simulink model "main"  (R2025a)
settings: Solver=VariableStepAuto  StartTime=0.0  StopTime=20  RelTol=1e-3
model workspace (MAT data in the model file):
  AccelNoise = [6.4e-07 6.4e-07 6.4e-07]
  AccelSampleTime = 0.001
  BaroSampleTime = 0.02
  BurnTime = 3.5
  GPSSampleTime = 0.06
  GimbalDelay = 0.02
  GimbalMaxRate = 5
  GimbalMaxSkew = 0.0872665
  Gravity = 9.81
  GyroNoise = [1.1e-08 1.1e-08 1.1e-08]
  GyroSampleTime = 0.001
  IMULocation = [0 0 0]
  InitialCG = [0 0 0]
  Mass = 1
  MaxAttitudeSetpoint = 0.15
  MaxThrust = 25
  MinThrust = 12
  MomentArm = 0.28
  RocketImpulse = 49.6
  RotationMatrix = [1  0  0; 0  1  0; 0  0  1]
  ServoSampleTime = 0.02
  Sig = Simulink.Signal
  Sig.Dimensions = -1
  Sig.DimensionsMode = 'auto'
  Sig.Complexity = 'auto'
  Sig.SampleTime = -1
  Sig.SamplingMode = 'auto'
  Sig.DataType = 'auto'
  Sig1 = Simulink.Signal
  Sig1.Dimensions = -1
  Sig1.DimensionsMode = 'auto'
  Sig1.Complexity = 'auto'
  Sig1.SampleTime = -1
  Sig1.SamplingMode = 'auto'
  Sig1.DataType = 'auto'
  VehicleMOI = [0.02  0  0; 0  0.1  0; 0  0  0.1]
  WheelDelay = 0.02
  WheelMOI = 0.0045
  WheelMaxAcceleration = 120
  WheelMaxRate = 500
  WheelSampleTime = 0.05
undefined symbols (not defined in the file): DiscIntNeverNeededParam
libraries: slpidlib x5, aerolibutil x4, aerolibnav x2, aerolibsim3d x2, sensorgpslib x1, sim3dlib x1, matrix_library x1
(part 1 of 2)
settings Model: Creator=jebid  LastModifiedBy=jebid

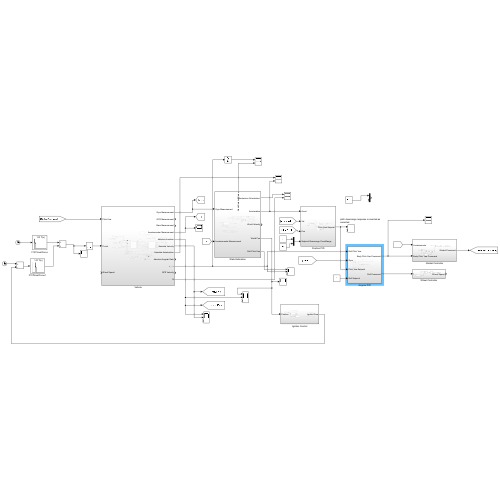
[thumbnail: Simulink's stored preview of the top-level diagram]
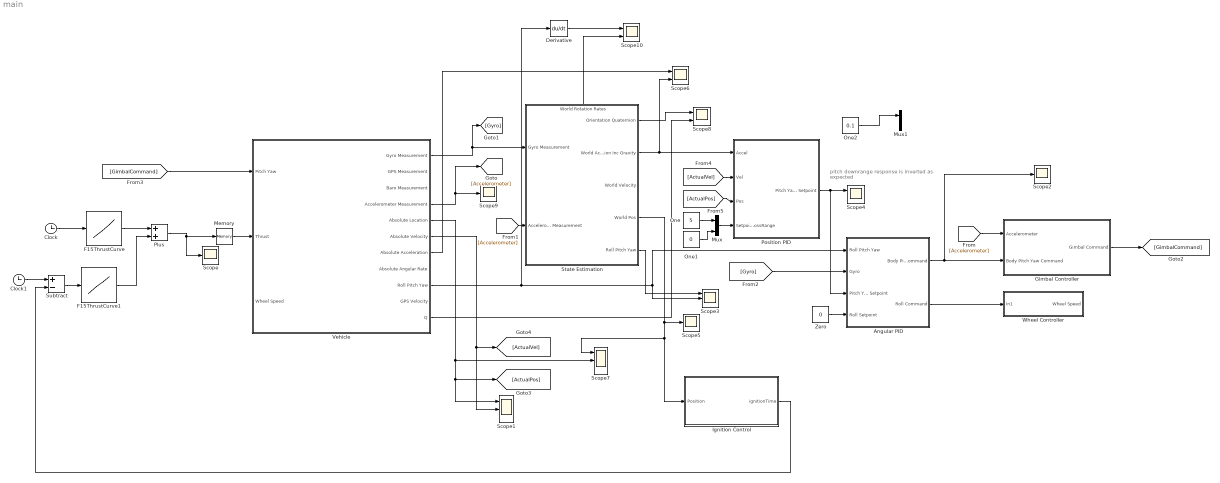
== system main ==
  note: pitch downrange response is inverted as expected
  Angular PID : Subsystem
  Clock : Clock
  Clock1 : Clock
  Derivative : Derivative
  F15ThrustCurve : Lookup_n-D  NumberOfTableDimensions=1  BreakpointsForDimension1=[0;0.14799999999999999;0.22800000000000001;0.29399999999999998;0.35299999999999998;0.38200000000000001;0.41899999999999998;0.47699999999999998;0.52000000000000002;0.59299999999999997;0.68799999999999994;0.85499999999999998;1.0369999999999999;1.2050000000000001;1.423;1.452;1.5029999999999999;1.736;1.9550000000000001;2.21;2.4940000000000002;2.7629999999999999;3.1200000000000001;3.3820000000000001;3.4039999999999999;3.4180000000000001;3.4500000000000002;30]  Table=[0;7.6379999999999999;12.253;16.390999999999998;20.210000000000001;22.756;25.260000000000002;23.074000000000002;20.844999999999999;19.093;17.5;16.225000000000001;15.427;14.948;14.627000000000001;15.741;14.785;14.622999999999999;14.303000000000001;14.141;13.819000000000001;13.337999999999999;13.334;13.013;9.3520000000000003;4.8949999999999996;0;0]  InternalRulePriority=Speed  RndMeth=Simplest
  F15ThrustCurve1 : Lookup_n-D  NumberOfTableDimensions=1  BreakpointsForDimension1=[-10;0;0.14799999999999999;0.22800000000000001;0.29399999999999998;0.35299999999999998;0.38200000000000001;0.41899999999999998;0.47699999999999998;0.52000000000000002;0.59299999999999997;0.68799999999999994;0.85499999999999998;1.0369999999999999;1.2050000000000001;1.423;1.452;1.5029999999999999;1.736;1.9550000000000001;2.21;2.4940000000000002;2.7629999999999999;3.1200000000000001;3.3820000000000001;3.4039999999999999;3.4180000000000001;3.4500000000000002;30]  Table=[0;0;7.6379999999999999;12.253;16.390999999999998;20.210000000000001;22.756;25.260000000000002;23.074000000000002;20.844999999999999;19.093;17.5;16.225000000000001;15.427;14.948;14.627000000000001;15.741;14.785;14.622999999999999;14.303000000000001;14.141;13.819000000000001;13.337999999999999;13.334;13.013;9.3520000000000003;4.8949999999999996;0;0]  InternalRulePriority=Speed  RndMeth=Simplest
  Gimbal Controller : Subsystem
  Ignition Control : Subsystem
  Memory : Memory
  Mux : Mux  Inputs=2
  Mux1 : Mux  Inputs=2
  One : Constant  Value=5  OutDataTypeStr=Inherit: Inherit via back propagation
  One1 : Constant  Value=0  OutDataTypeStr=Inherit: Inherit via back propagation
  One2 : Constant  Value=0.1  OutDataTypeStr=Inherit: Inherit via back propagation
  Plus : Sum
  Position PID : Subsystem
  Scope{,2,5,9} (4 alike) : Scope
      Scope settings: ActiveDisplayYMinimum=-50.736387173772314  ActiveDisplayYMaximum=31.586324733859495  DataLoggingVariableName=ScopeData4
      Scope2 settings: ActiveDisplayYMinimum=-0.14523916731500583  ActiveDisplayYMaximum=0.12648126595285003  DataLoggingVariableName=ScopeData6
      Scope5 settings: ActiveDisplayYMinimum=-31.391925729370655  ActiveDisplayYMaximum=52.800871093838978  DataLoggingVariableName=ScopeData8
      Scope9 settings: ActiveDisplayYMinimum=-1  ActiveDisplayYMaximum=1  DataLoggingVariableName=ScopeData27
  Scope1 : Scope  NumInputPorts=3
      settings: ActiveDisplayYMinimum=-22.683231133577891  ActiveDisplayYMaximum=11.292289740871924  DataLoggingVariableName=ScopeData5
  Scope{4,6,8,10} (4 alike) : Scope  NumInputPorts=2
      Scope10 settings: ActiveDisplayYMinimum=0.0077606363117146  ActiveDisplayYMaximum=0.18302244133274109  DataLoggingVariableName=ScopeData29
      Scope4 settings: ActiveDisplayYMinimum=-0.36702058756794975  ActiveDisplayYMaximum=0.56051213237813946  DataLoggingVariableName=ScopeData14
      Scope6 settings: ActiveDisplayYMinimum=-12.621728801475598  ActiveDisplayYMaximum=24.903102267700667  DataLoggingVariableName=ScopeData15
      Scope8 settings: ActiveDisplayYMinimum=0.705787790554492  ActiveDisplayYMaximum=0.96095471743838046  DataLoggingVariableName=ScopeData17
  Scope3 : Scope  NumInputPorts=3
      settings: ActiveDisplayYMinimum=-0.2363689882566378  ActiveDisplayYMaximum=0.3544136524668004  DataLoggingVariableName=ScopeData7
  Scope7 : Scope  NumInputPorts=3
      settings: ActiveDisplayYMinimum=-22.879561375629812  ActiveDisplayYMaximum=31.102735527921809  DataLoggingVariableName=ScopeData16
  State Estimation : Subsystem
      settings: PortSchema="{\"entries\":[{\"content\":{\"sides\":[{\"content\":{\"connectorIds\":[\"In1\",\"In2\"]},\"type\":\"ConnectorPlacement.EquallySpacedRectSide\",\"uuid\":\"2c2c3dca-e4ed-4564-ae6f-11a940ebc0d2\"},{\"content\":{\"connectorIds\":[\"Out1\",\"Out2\",\"Out3\",\"Out4\",\"Out5\"],\"side\":\"RIGHT\"},\"type\":\"ConnectorPlacement.EquallySpacedRectSide\",\"uuid\":\"8d125d98-ae45-4016-ae84-ebbc5244d165\"},{\"content\":{\"connectorIds\":[\"Out6\"],\"side\":\"TOP\"},\"type\":\"ConnectorPlacement.EquallySpacedRectSide\",\"uuid\":\"d438488b-91d6-49f1-8b44-fd6b40ea1e09\"}]},\"type\":\"ConnectorPlacement.EquallySpacedConnector\",\"uuid\":\"85e5d060-1813-434d-86b8-3131fa751346\"}],\"packageUris\":[\"http://schema.mathworks.com/mf0/Connector/R2020b\"],\"version\":\"1.0\"}"
  Subtract : Sum  Inputs=+-
  Vehicle : Subsystem
  Wheel Controller : Subsystem
  Zero : Constant  Value=0  OutDataTypeStr=Inherit: Inherit via back propagation
  wires:
  Clock/1 -> F15ThrustCurve/1
  Vehicle/1(Gyro Measurement) -> [Gyro], State Estimation/1(Gyro Measurement)
  State Estimation/4(World Pos) -> Scope5/1, Ignition Control/1(Position), Scope7/1
  F15ThrustCurve/1 -> Plus/1
  Plus/1 -> Scope/1, Memory/1
  Clock1/1 -> Subtract/1
  Ignition Control/1(ignitionTime) -> Subtract/2
  Subtract/1 -> F15ThrustCurve1/1
  F15ThrustCurve1/1 -> Plus/2
  State Estimation/2(World Acceleration Inc Gravity) -> Scope6/2, Position PID/1(Accel)
  Zero/1 -> Angular PID/4(Roll Setpoint)
  Angular PID/2(Roll Command) -> Wheel Controller/1(In1)
  Vehicle/4(Accelerometer Measurement) -> Scope9/1, [Accelerometer]
  [Accelerometer] -> Gimbal Controller/1(Accelerometer)
  [Accelerometer] -> State Estimation/2(Accelerometer Measurement)
  [Gyro] -> Angular PID/2(Gyro)
  Gimbal Controller/1(Gimbal Command) -> [GimbalCommand]
  Position PID/1(Pitch Yaw Setpoint) -> Angular PID/3(Pitch Yaw Setpoint), Scope4/1
  Vehicle/5(Absolute Location) -> Scope7/2, [ActualPos], Scope1/1
  Mux/1 -> Position PID/4(Setpoint Downrange CrossRange)
  One/1 -> Mux/1
  One1/1 -> Mux/2
  Vehicle/7(Absolute Acceleration) -> Scope6/1
  Vehicle/6(Absolute Velocity) -> [ActualVel], Scope1/2
  [ActualVel] -> Position PID/2(Vel)
  [ActualPos] -> Position PID/3(Pos)
  State Estimation/5(Roll Pitch Yaw) -> Scope3/1
  State Estimation/1(Orientation Quaternion) -> Scope8/1
  Vehicle/11(Q) -> Scope8/2
  Memory/1 -> Vehicle/2(Thrust)
  [GimbalCommand] -> Vehicle/1(Pitch Yaw)
  Angular PID/1(Body Pitch Yaw Command) -> Scope2/1, Gimbal Controller/2(Body Pitch Yaw Command)
  State Estimation/6(World Rotation Rates) -> Scope10/2
  Derivative/1 -> Scope10/1
  Vehicle/9(Roll Pitch Yaw) -> Derivative/1, Scope3/2, Angular PID/1(Roll Pitch Yaw)
  One2/1 -> Mux1/1

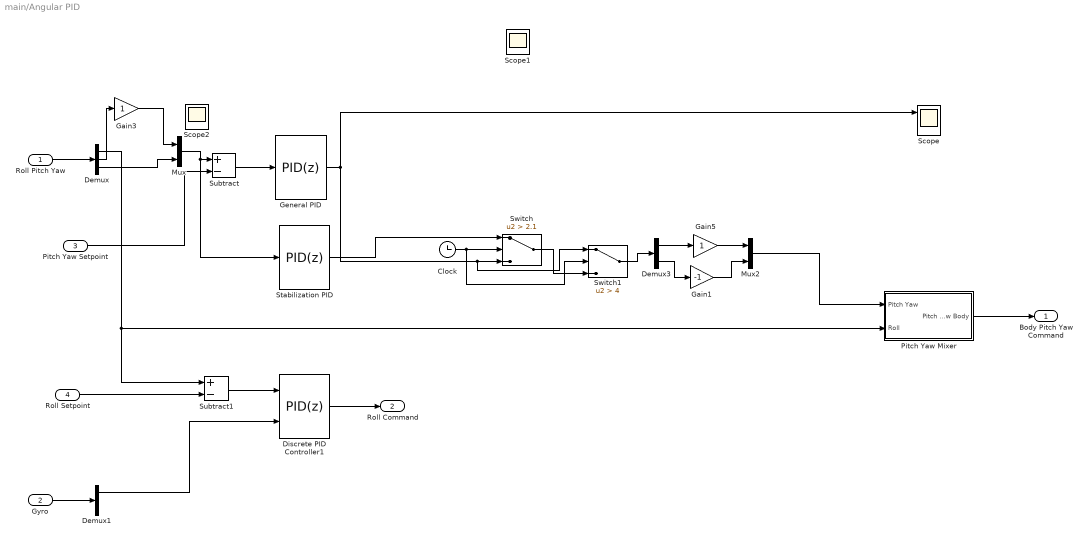
== system main/Angular PID ==
  Roll Pitch Yaw : Inport
  Gyro : Inport  Port=2
  Pitch Yaw Setpoint : Inport  Port=3
  Roll Setpoint : Inport  Port=4
  Clock : Clock
  Demux : Demux  Outputs=3
  Demux1 : Demux  Outputs=3
  Demux3 : Demux  Outputs=2
  Discrete PID Controller1 : slpidlib/PID Controller  Controller=PID  Form=Parallel  TimeDomain=Discrete-time  UseExternalTs=off  SampleTime=0.01  IntegratorMethod=Forward Euler  FilterMethod=Forward Euler  ControllerParametersSource=internal  P=0.05  I=0  UseKiTs=on  D=-0.1  UseExternalDerivativeSource=on  N=100  UseFilter=on  TunerSelectOption=Transfer Function Based (PID Tuner App)  InitialConditionSource=internal  InitialConditionForIntegrator=0  InitialConditionForFilter=0  DifferentiatorICPrevScaledInput=0  ExternalReset=none  TrackingMode=off  Kt=1  LimitOutput=off  SatLimitsSource=internal  UpperSaturationLimit=inf  LowerSaturationLimit=-inf  LinearizeAsGain=off  AntiWindupMode=none  Kb=1  LimitIntegrator=off  UpperIntegratorSaturationLimit=inf  LowerIntegratorSaturationLimit=-inf  POutMin=[]  POutMax=[]  IOutMin=[]  IOutMax=[]  DOutMin=[]  DOutMax=[]  NOutMin=[]  NOutMax=[]  SumOutMin=[]  SumOutMax=[]  SaturationOutMin=[]  SaturationOutMax=[]  PParamMin=[]  PParamMax=[]  IParamMin=[]  IParamMax=[]  DParamMin=[]  DParamMax=[]  NParamMin=[]  NParamMax=[]  KbParamMin=[]  KbParamMax=[]  KtParamMin=[]  KtParamMax=[]  KbOutMin=[]  KbOutMax=[]  KtOutMin=[]  KtOutMax=[]  IntegratorOutMin=[]  IntegratorOutMax=[]  FilterOutMin=[]  FilterOutMax=[]  SumI1OutMin=[]  SumI1OutMax=[]  SumI2OutMin=[]  SumI2OutMax=[]  SumI3OutMin=[]  SumI3OutMax=[]  SumI4OutMin=[]  SumI4OutMax=[]  SumDOutMin=[]  SumDOutMax=[]  DifferentiatorOutMin=[]  DifferentiatorOutMax=[]  FilterDiffOutCoefMin=[]  FilterDiffOutCoefMax=[]  ReciprocalOutMin=[]  ReciprocalOutMax=[]  SumDenOutMin=[]  SumDenOutMax=[]  SumNumOutMin=[]  SumNumOutMax=[]  DivideOutMin=[]  DivideOutMax=[]  UdiffTsProdOutMin=[]  UdiffTsProdOutMax=[]  NTsProdOutMin=[]  NTsProdOutMax=[]  UintegralTsProdOutMin=[]  UintegralTsProdOutMax=[]  UngainTsProdOutMin=[]  UngainTsProdOutMax=[]  ClampingZeroOutDataTypeStr=Inherit: Inherit via back propagation  ClampingZeroOutMin=[]  ClampingZeroOutMax=[]  FilterDenConstantOutDataTypeStr=Inherit: Inherit via back propagation  FilterDenConstantOutMin=[]  FilterDenConstantOutMax=[]  PCopyOutDataTypeStr=Inherit: Inherit via back propagation  PCopyOutMin=[]  PCopyOutMax=[]  NCopyOutDataTypeStr=Inherit: Inherit via back propagation  NCopyOutMin=[]  NCopyOutMax=[]  IntegratorContinuousStateAttributes=''  IntegratorStateMustResolveToSignalObject=off  IntegratorRTWStateStorageClass=Auto  FilterContinuousStateAttributes=''  FilterStateMustResolveToSignalObject=off  FilterRTWStateStorageClass=Auto  ParallelPVariant=InternalParameters  IdealPVariant=Disabled  IVariant=InternalParameters  DVariant=InternalParameters  IntegratorVariant=Discrete  SatVariant=Disabled  AWVariant=Passthrough  PCopyVariant=Disabled  TRVariant=Disabled  FdbkBlocksVariant=Forward  IdealPFdbkVariant=Disabled  SatFdbkVariant=Disabled  DerivativeFilterVariant=ForwardEulerFilterOnly  NVariant=InternalParameters  NCopyVariant=Disabled  FilterICVariant=InternalICsFilter  IntegratorICVariant=InternalICs  ExternalResetVariant=Disabled  TRSumVariant=Passthrough  SumFdbkVariant=Disabled  SumVariant=Sum_PID  TsampFilterVariant=InternalTs  TsampNgainVariant=Passthrough  TsampIntegralVariant=Disabled_SignalSpec  ExternalSaturationOutDataTypeStr=Inherit: Same as second input  DerivativeSourceVariant=ExternalYdot  PreIntVariant=InternalPreInt
      settings: LibrarySourceBlock=simulink/Discrete/Discrete PID Controller
  Gain1 : Gain  Gain=-1
  Gain3 : Gain
  Gain5 : Gain
  General PID : slpidlib/PID Controller  Controller=PID  Form=Parallel  TimeDomain=Discrete-time  UseExternalTs=off  SampleTime=0.01  IntegratorMethod=Forward Euler  FilterMethod=Forward Euler  ControllerParametersSource=internal  P=-0.9  I=0  UseKiTs=on  D=-0.3  UseExternalDerivativeSource=off  N=100  UseFilter=on  TunerSelectOption=Transfer Function Based (PID Tuner App)  InitialConditionSource=internal  InitialConditionForIntegrator=0  InitialConditionForFilter=0  DifferentiatorICPrevScaledInput=0  ExternalReset=none  TrackingMode=off  Kt=1  LimitOutput=off  SatLimitsSource=internal  UpperSaturationLimit=inf  LowerSaturationLimit=-inf  LinearizeAsGain=off  AntiWindupMode=none  Kb=1  LimitIntegrator=off  UpperIntegratorSaturationLimit=inf  LowerIntegratorSaturationLimit=-inf  POutMin=[]  POutMax=[]  IOutMin=[]  IOutMax=[]  DOutMin=[]  DOutMax=[]  NOutMin=[]  NOutMax=[]  SumOutMin=[]  SumOutMax=[]  SaturationOutMin=[]  SaturationOutMax=[]  PParamMin=[]  PParamMax=[]  IParamMin=[]  IParamMax=[]  DParamMin=[]  DParamMax=[]  NParamMin=[]  NParamMax=[]  KbParamMin=[]  KbParamMax=[]  KtParamMin=[]  KtParamMax=[]  KbOutMin=[]  KbOutMax=[]  KtOutMin=[]  KtOutMax=[]  IntegratorOutMin=[]  IntegratorOutMax=[]  FilterOutMin=[]  FilterOutMax=[]  SumI1OutMin=[]  SumI1OutMax=[]  SumI2OutMin=[]  SumI2OutMax=[]  SumI3OutMin=[]  SumI3OutMax=[]  SumI4OutMin=[]  SumI4OutMax=[]  SumDOutMin=[]  SumDOutMax=[]  DifferentiatorOutMin=[]  DifferentiatorOutMax=[]  FilterDiffOutCoefMin=[]  FilterDiffOutCoefMax=[]  ReciprocalOutMin=[]  ReciprocalOutMax=[]  SumDenOutMin=[]  SumDenOutMax=[]  SumNumOutMin=[]  SumNumOutMax=[]  DivideOutMin=[]  DivideOutMax=[]  UdiffTsProdOutMin=[]  UdiffTsProdOutMax=[]  NTsProdOutMin=[]  NTsProdOutMax=[]  UintegralTsProdOutMin=[]  UintegralTsProdOutMax=[]  UngainTsProdOutMin=[]  UngainTsProdOutMax=[]  ClampingZeroOutDataTypeStr=Inherit: Inherit via back propagation  ClampingZeroOutMin=[]  ClampingZeroOutMax=[]  FilterDenConstantOutDataTypeStr=Inherit: Inherit via back propagation  FilterDenConstantOutMin=[]  FilterDenConstantOutMax=[]  PCopyOutDataTypeStr=Inherit: Inherit via back propagation  PCopyOutMin=[]  PCopyOutMax=[]  NCopyOutDataTypeStr=Inherit: Inherit via back propagation  NCopyOutMin=[]  NCopyOutMax=[]  IntegratorContinuousStateAttributes=''  IntegratorStateMustResolveToSignalObject=off  IntegratorRTWStateStorageClass=Auto  FilterContinuousStateAttributes=''  FilterStateMustResolveToSignalObject=off  FilterRTWStateStorageClass=Auto  ParallelPVariant=InternalParameters  IdealPVariant=Disabled  IVariant=InternalParameters  DVariant=InternalParameters  IntegratorVariant=Discrete  SatVariant=Disabled  AWVariant=Passthrough  PCopyVariant=Disabled  TRVariant=Disabled  FdbkBlocksVariant=Forward  IdealPFdbkVariant=Disabled  SatFdbkVariant=Disabled  DerivativeFilterVariant=ForwardEulerFilter  NVariant=InternalParameters  NCopyVariant=Disabled  FilterICVariant=InternalICsFilter  IntegratorICVariant=InternalICs  ExternalResetVariant=Disabled  TRSumVariant=Passthrough  SumFdbkVariant=Disabled  SumVariant=Sum_PID  TsampFilterVariant=InternalTs  TsampNgainVariant=Passthrough  TsampIntegralVariant=Disabled_SignalSpec  ExternalSaturationOutDataTypeStr=Inherit: Same as second input  DerivativeSourceVariant=ErrorSignal  PreIntVariant=InternalPreInt
      settings: LibrarySourceBlock=simulink/Discrete/Discrete PID Controller
  Mux : Mux  Inputs=2
  Mux2 : Mux  Inputs=2
  Pitch Yaw Mixer : Subsystem
  Scope : Scope  NumInputPorts=2
      settings: ActiveDisplayYMinimum=-0.39866563358143736  ActiveDisplayYMaximum=0.45737889252656044  DataLoggingVariableName=ScopeData9
  Scope1 : Scope
      settings: ActiveDisplayYMinimum=-0.518033395212612  ActiveDisplayYMaximum=0.97602188870445683  DataLoggingVariableName=ScopeData28
  Scope2 : Scope
      settings: ActiveDisplayYMinimum=-0.36095317144892464  ActiveDisplayYMaximum=0.65877109038905879  DataLoggingVariableName=ScopeData12
  Stabilization PID : slpidlib/PID Controller  Controller=PID  Form=Parallel  TimeDomain=Discrete-time  UseExternalTs=off  SampleTime=0.01  IntegratorMethod=Forward Euler  FilterMethod=Forward Euler  ControllerParametersSource=internal  P=-0.9  I=0  UseKiTs=on  D=-0.3  UseExternalDerivativeSource=off  N=100  UseFilter=on  TunerSelectOption=Transfer Function Based (PID Tuner App)  InitialConditionSource=internal  InitialConditionForIntegrator=0  InitialConditionForFilter=0  DifferentiatorICPrevScaledInput=0  ExternalReset=none  TrackingMode=off  Kt=1  LimitOutput=off  SatLimitsSource=internal  UpperSaturationLimit=inf  LowerSaturationLimit=-inf  LinearizeAsGain=off  AntiWindupMode=none  Kb=1  LimitIntegrator=off  UpperIntegratorSaturationLimit=inf  LowerIntegratorSaturationLimit=-inf  POutMin=[]  POutMax=[]  IOutMin=[]  IOutMax=[]  DOutMin=[]  DOutMax=[]  NOutMin=[]  NOutMax=[]  SumOutMin=[]  SumOutMax=[]  SaturationOutMin=[]  SaturationOutMax=[]  PParamMin=[]  PParamMax=[]  IParamMin=[]  IParamMax=[]  DParamMin=[]  DParamMax=[]  NParamMin=[]  NParamMax=[]  KbParamMin=[]  KbParamMax=[]  KtParamMin=[]  KtParamMax=[]  KbOutMin=[]  KbOutMax=[]  KtOutMin=[]  KtOutMax=[]  IntegratorOutMin=[]  IntegratorOutMax=[]  FilterOutMin=[]  FilterOutMax=[]  SumI1OutMin=[]  SumI1OutMax=[]  SumI2OutMin=[]  SumI2OutMax=[]  SumI3OutMin=[]  SumI3OutMax=[]  SumI4OutMin=[]  SumI4OutMax=[]  SumDOutMin=[]  SumDOutMax=[]  DifferentiatorOutMin=[]  DifferentiatorOutMax=[]  FilterDiffOutCoefMin=[]  FilterDiffOutCoefMax=[]  ReciprocalOutMin=[]  ReciprocalOutMax=[]  SumDenOutMin=[]  SumDenOutMax=[]  SumNumOutMin=[]  SumNumOutMax=[]  DivideOutMin=[]  DivideOutMax=[]  UdiffTsProdOutMin=[]  UdiffTsProdOutMax=[]  NTsProdOutMin=[]  NTsProdOutMax=[]  UintegralTsProdOutMin=[]  UintegralTsProdOutMax=[]  UngainTsProdOutMin=[]  UngainTsProdOutMax=[]  ClampingZeroOutDataTypeStr=Inherit: Inherit via back propagation  ClampingZeroOutMin=[]  ClampingZeroOutMax=[]  FilterDenConstantOutDataTypeStr=Inherit: Inherit via back propagation  FilterDenConstantOutMin=[]  FilterDenConstantOutMax=[]  PCopyOutDataTypeStr=Inherit: Inherit via back propagation  PCopyOutMin=[]  PCopyOutMax=[]  NCopyOutDataTypeStr=Inherit: Inherit via back propagation  NCopyOutMin=[]  NCopyOutMax=[]  IntegratorContinuousStateAttributes=''  IntegratorStateMustResolveToSignalObject=off  IntegratorRTWStateStorageClass=Auto  FilterContinuousStateAttributes=''  FilterStateMustResolveToSignalObject=off  FilterRTWStateStorageClass=Auto  ParallelPVariant=InternalParameters  IdealPVariant=Disabled  IVariant=InternalParameters  DVariant=InternalParameters  IntegratorVariant=Discrete  SatVariant=Disabled  AWVariant=Passthrough  PCopyVariant=Disabled  TRVariant=Disabled  FdbkBlocksVariant=Forward  IdealPFdbkVariant=Disabled  SatFdbkVariant=Disabled  DerivativeFilterVariant=ForwardEulerFilter  NVariant=InternalParameters  NCopyVariant=Disabled  FilterICVariant=InternalICsFilter  IntegratorICVariant=InternalICs  ExternalResetVariant=Disabled  TRSumVariant=Passthrough  SumFdbkVariant=Disabled  SumVariant=Sum_PID  TsampFilterVariant=InternalTs  TsampNgainVariant=Passthrough  TsampIntegralVariant=Disabled_SignalSpec  ExternalSaturationOutDataTypeStr=Inherit: Same as second input  DerivativeSourceVariant=ErrorSignal  PreIntVariant=InternalPreInt
      settings: LibrarySourceBlock=simulink/Discrete/Discrete PID Controller
  Subtract : Sum  Inputs=+-
  Subtract1 : Sum  Inputs=+-
  Switch : Switch  Criteria=u2 > Threshold  Threshold=2.1  SaturateOnIntegerOverflow=off  InputSameDT=off
  Switch1 : Switch  Criteria=u2 > Threshold  Threshold=4  SaturateOnIntegerOverflow=off  InputSameDT=off
  Body Pitch Yaw Command : Outport
  Roll Command : Outport  Port=2
  wires:
  Roll Pitch Yaw/1 -> Demux/1
  Gyro/1 -> Demux1/1
  Mux/1 -> Stabilization PID/1, Subtract/1
  Pitch Yaw Setpoint/1 -> Subtract/2
  Subtract1/1 -> Discrete PID Controller1/1
  Roll Setpoint/1 -> Subtract1/2
  Discrete PID Controller1/1 -> Roll Command/1
  Clock/1 -> Switch1/2, Switch/2
  Switch/1 -> Switch1/3
  Subtract/1 -> General PID/1
  General PID/1 -> Switch1/1, Switch/3, Scope/1
  Pitch Yaw Mixer/1(Pitch Yaw Body) -> Body Pitch Yaw Command/1
  Demux1/1 -> Discrete PID Controller1/2
  Demux/2 -> Gain3/1
  Demux/3 -> Mux/2
  Demux/1 -> Subtract1/1, Pitch Yaw Mixer/2(Roll)
  Gain3/1 -> Mux/1
  Stabilization PID/1 -> Switch/1
  Demux3/1 -> Gain5/1
  Gain5/1 -> Mux2/1
  Gain1/1 -> Mux2/2
  Demux3/2 -> Gain1/1
  Switch1/1 -> Demux3/1
  Mux2/1 -> Pitch Yaw Mixer/1(Pitch Yaw)

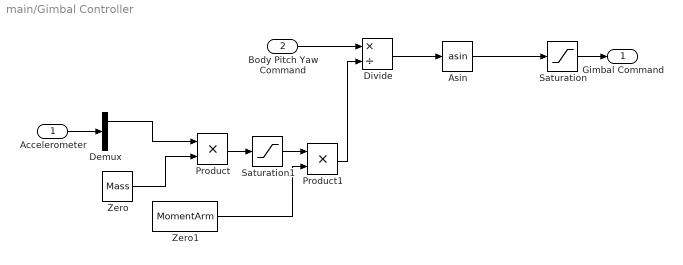
== system main/Gimbal Controller ==
  Accelerometer : Inport
  Body Pitch Yaw Command : Inport  Port=2
  Asin : Trigonometry  Operator=asin
  Demux : Demux  Outputs=3
  Divide : Product  Inputs=*/
  Product : Product
  Product1 : Product
  Saturation : Saturate  UpperLimit=GimbalMaxSkew  LowerLimit=-GimbalMaxSkew
  Saturation1 : Saturate  UpperLimit=MaxThrust  LowerLimit=MinThrust
  Zero : Constant  Value=Mass  OutDataTypeStr=Inherit: Inherit via back propagation
  Zero1 : Constant  Value=MomentArm  OutDataTypeStr=Inherit: Inherit via back propagation
  Gimbal Command : Outport
  wires:
  Saturation/1 -> Gimbal Command/1
  Accelerometer/1 -> Demux/1
  Body Pitch Yaw Command/1 -> Divide/1
  Zero/1 -> Product/2
  Product/1 -> Saturation1/1
  Saturation1/1 -> Product1/1
  Zero1/1 -> Product1/2
  Product1/1 -> Divide/2
  Divide/1 -> Asin/1
  Asin/1 -> Saturation/1
  Demux/1 -> Product/1

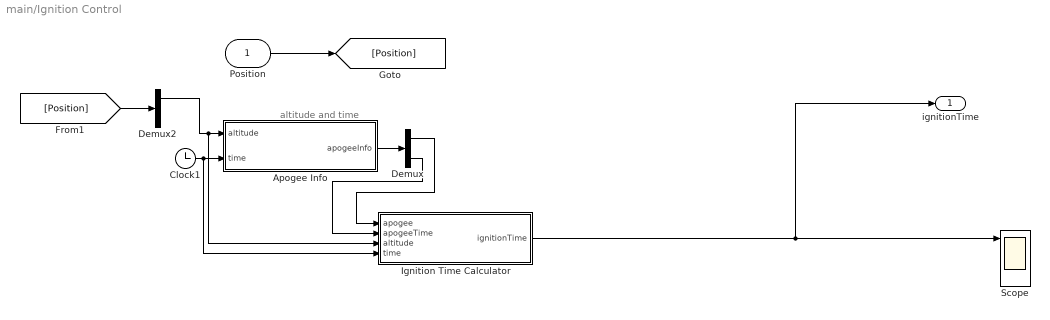
== system main/Ignition Control ==
  note: altitude and time
  Position : Inport
  Apogee Info : MATLAB Function  TreatAsAtomicUnit=on
  Clock1 : Clock
  Demux : Demux  Outputs=2
  Demux2 : Demux  Outputs=3
  Ignition Time Calculator : MATLAB Function  TreatAsAtomicUnit=on
  Scope : Scope  NumInputPorts=3
      settings: ActiveDisplayYMinimum=-11.611282648823959  ActiveDisplayYMaximum=65.175222226116219  DataLoggingVariableName=ScopeData3
  ignitionTime : Outport
  wires:
  Apogee Info/1(apogeeInfo) -> Demux/1
  Position/1 -> [Position]
  [Position] -> Demux2/1
  Clock1/1 -> Ignition Time Calculator/4(time), Apogee Info/2(time)
  Demux/1 -> Ignition Time Calculator/1(apogee)
  Ignition Time Calculator/1(ignitionTime) -> ignitionTime/1, Scope/1
  Demux/2 -> Ignition Time Calculator/2(apogeeTime)
  Demux2/1 -> Ignition Time Calculator/3(altitude), Apogee Info/1(altitude)

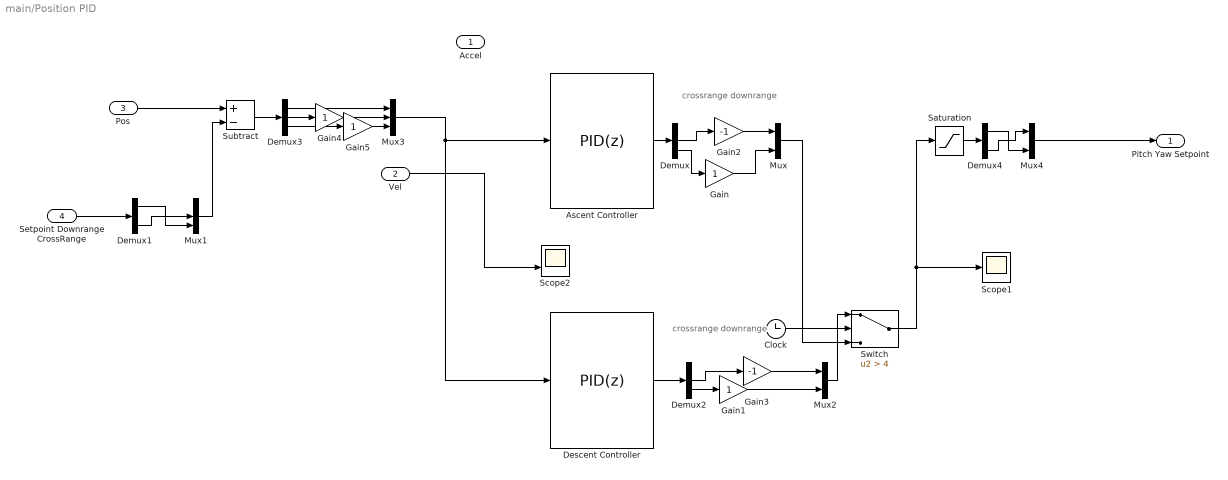
== system main/Position PID ==
  note: crossrange downrange
  note: crossrange downrange
  Accel : Inport
  Vel : Inport  Port=2
  Pos : Inport  Port=3
  Setpoint Downrange CrossRange : Inport  Port=4
  Ascent Controller : slpidlib/PID Controller  Controller=PID  Form=Parallel  TimeDomain=Discrete-time  UseExternalTs=off  SampleTime=-1  IntegratorMethod=Forward Euler  FilterMethod=Forward Euler  ControllerParametersSource=internal  P=0.065  I=0  UseKiTs=on  D=0.3  UseExternalDerivativeSource=off  N=100  UseFilter=on  TunerSelectOption=Transfer Function Based (PID Tuner App)  InitialConditionSource=internal  InitialConditionForIntegrator=0  InitialConditionForFilter=0  DifferentiatorICPrevScaledInput=0  ExternalReset=none  TrackingMode=off  Kt=1  LimitOutput=off  SatLimitsSource=internal  UpperSaturationLimit=inf  LowerSaturationLimit=-inf  LinearizeAsGain=off  AntiWindupMode=none  Kb=1  LimitIntegrator=off  UpperIntegratorSaturationLimit=inf  LowerIntegratorSaturationLimit=-inf  POutMin=[]  POutMax=[]  IOutMin=[]  IOutMax=[]  DOutMin=[]  DOutMax=[]  NOutMin=[]  NOutMax=[]  SumOutMin=[]  SumOutMax=[]  SaturationOutMin=[]  SaturationOutMax=[]  PParamMin=[]  PParamMax=[]  IParamMin=[]  IParamMax=[]  DParamMin=[]  DParamMax=[]  NParamMin=[]  NParamMax=[]  KbParamMin=[]  KbParamMax=[]  KtParamMin=[]  KtParamMax=[]  KbOutMin=[]  KbOutMax=[]  KtOutMin=[]  KtOutMax=[]  IntegratorOutMin=[]  IntegratorOutMax=[]  FilterOutMin=[]  FilterOutMax=[]  SumI1OutMin=[]  SumI1OutMax=[]  SumI2OutMin=[]  SumI2OutMax=[]  SumI3OutMin=[]  SumI3OutMax=[]  SumI4OutMin=[]  SumI4OutMax=[]  SumDOutMin=[]  SumDOutMax=[]  DifferentiatorOutMin=[]  DifferentiatorOutMax=[]  FilterDiffOutCoefMin=[]  FilterDiffOutCoefMax=[]  ReciprocalOutMin=[]  ReciprocalOutMax=[]  SumDenOutMin=[]  SumDenOutMax=[]  SumNumOutMin=[]  SumNumOutMax=[]  DivideOutMin=[]  DivideOutMax=[]  UdiffTsProdOutMin=[]  UdiffTsProdOutMax=[]  NTsProdOutMin=[]  NTsProdOutMax=[]  UintegralTsProdOutMin=[]  UintegralTsProdOutMax=[]  UngainTsProdOutMin=[]  UngainTsProdOutMax=[]  ClampingZeroOutDataTypeStr=Inherit: Inherit via back propagation  ClampingZeroOutMin=[]  ClampingZeroOutMax=[]  FilterDenConstantOutDataTypeStr=Inherit: Inherit via back propagation  FilterDenConstantOutMin=[]  FilterDenConstantOutMax=[]  PCopyOutDataTypeStr=Inherit: Inherit via back propagation  PCopyOutMin=[]  PCopyOutMax=[]  NCopyOutDataTypeStr=Inherit: Inherit via back propagation  NCopyOutMin=[]  NCopyOutMax=[]  IntegratorContinuousStateAttributes=''  IntegratorStateMustResolveToSignalObject=off  IntegratorRTWStateStorageClass=Auto  FilterContinuousStateAttributes=''  FilterStateMustResolveToSignalObject=off  FilterRTWStateStorageClass=Auto  ParallelPVariant=InternalParameters  IdealPVariant=Disabled  IVariant=InternalParameters  DVariant=InternalParameters  IntegratorVariant=Discrete  SatVariant=Disabled  AWVariant=Passthrough  PCopyVariant=Disabled  TRVariant=Disabled  FdbkBlocksVariant=Forward  IdealPFdbkVariant=Disabled  SatFdbkVariant=Disabled  DerivativeFilterVariant=ForwardEulerFilter  NVariant=InternalParameters  NCopyVariant=Disabled  FilterICVariant=InternalICsFilter  IntegratorICVariant=InternalICs  ExternalResetVariant=Disabled  TRSumVariant=Passthrough  SumFdbkVariant=Disabled  SumVariant=Sum_PID  TsampFilterVariant=InternalTs  TsampNgainVariant=Passthrough  TsampIntegralVariant=Disabled_SignalSpec  ExternalSaturationOutDataTypeStr=Inherit: Same as second input  DerivativeSourceVariant=ErrorSignal  PreIntVariant=InternalPreInt
      settings: LibrarySourceBlock=simulink/Discrete/Discrete PID Controller
  Clock : Clock
  Demux : Demux  Outputs=3
  Demux1 : Demux  Outputs=2
  Demux2 : Demux  Outputs=3
  Demux3 : Demux  Outputs=3
  Demux4 : Demux  Outputs=2
  Descent Controller : slpidlib/PID Controller  Controller=PID  Form=Parallel  TimeDomain=Discrete-time  UseExternalTs=off  SampleTime=-1  IntegratorMethod=Forward Euler  FilterMethod=Forward Euler  ControllerParametersSource=internal  P=0.065  I=0  UseKiTs=on  D=0.2  UseExternalDerivativeSource=off  N=100  UseFilter=on  TunerSelectOption=Transfer Function Based (PID Tuner App)  InitialConditionSource=internal  InitialConditionForIntegrator=0  InitialConditionForFilter=0  DifferentiatorICPrevScaledInput=0  ExternalReset=none  TrackingMode=off  Kt=1  LimitOutput=off  SatLimitsSource=internal  UpperSaturationLimit=inf  LowerSaturationLimit=-inf  LinearizeAsGain=off  AntiWindupMode=none  Kb=1  LimitIntegrator=off  UpperIntegratorSaturationLimit=inf  LowerIntegratorSaturationLimit=-inf  POutMin=[]  POutMax=[]  IOutMin=[]  IOutMax=[]  DOutMin=[]  DOutMax=[]  NOutMin=[]  NOutMax=[]  SumOutMin=[]  SumOutMax=[]  SaturationOutMin=[]  SaturationOutMax=[]  PParamMin=[]  PParamMax=[]  IParamMin=[]  IParamMax=[]  DParamMin=[]  DParamMax=[]  NParamMin=[]  NParamMax=[]  KbParamMin=[]  KbParamMax=[]  KtParamMin=[]  KtParamMax=[]  KbOutMin=[]  KbOutMax=[]  KtOutMin=[]  KtOutMax=[]  IntegratorOutMin=[]  IntegratorOutMax=[]  FilterOutMin=[]  FilterOutMax=[]  SumI1OutMin=[]  SumI1OutMax=[]  SumI2OutMin=[]  SumI2OutMax=[]  SumI3OutMin=[]  SumI3OutMax=[]  SumI4OutMin=[]  SumI4OutMax=[]  SumDOutMin=[]  SumDOutMax=[]  DifferentiatorOutMin=[]  DifferentiatorOutMax=[]  FilterDiffOutCoefMin=[]  FilterDiffOutCoefMax=[]  ReciprocalOutMin=[]  ReciprocalOutMax=[]  SumDenOutMin=[]  SumDenOutMax=[]  SumNumOutMin=[]  SumNumOutMax=[]  DivideOutMin=[]  DivideOutMax=[]  UdiffTsProdOutMin=[]  UdiffTsProdOutMax=[]  NTsProdOutMin=[]  NTsProdOutMax=[]  UintegralTsProdOutMin=[]  UintegralTsProdOutMax=[]  UngainTsProdOutMin=[]  UngainTsProdOutMax=[]  ClampingZeroOutDataTypeStr=Inherit: Inherit via back propagation  ClampingZeroOutMin=[]  ClampingZeroOutMax=[]  FilterDenConstantOutDataTypeStr=Inherit: Inherit via back propagation  FilterDenConstantOutMin=[]  FilterDenConstantOutMax=[]  PCopyOutDataTypeStr=Inherit: Inherit via back propagation  PCopyOutMin=[]  PCopyOutMax=[]  NCopyOutDataTypeStr=Inherit: Inherit via back propagation  NCopyOutMin=[]  NCopyOutMax=[]  IntegratorContinuousStateAttributes=''  IntegratorStateMustResolveToSignalObject=off  IntegratorRTWStateStorageClass=Auto  FilterContinuousStateAttributes=''  FilterStateMustResolveToSignalObject=off  FilterRTWStateStorageClass=Auto  ParallelPVariant=InternalParameters  IdealPVariant=Disabled  IVariant=InternalParameters  DVariant=InternalParameters  IntegratorVariant=Discrete  SatVariant=Disabled  AWVariant=Passthrough  PCopyVariant=Disabled  TRVariant=Disabled  FdbkBlocksVariant=Forward  IdealPFdbkVariant=Disabled  SatFdbkVariant=Disabled  DerivativeFilterVariant=ForwardEulerFilter  NVariant=InternalParameters  NCopyVariant=Disabled  FilterICVariant=InternalICsFilter  IntegratorICVariant=InternalICs  ExternalResetVariant=Disabled  TRSumVariant=Passthrough  SumFdbkVariant=Disabled  SumVariant=Sum_PID  TsampFilterVariant=InternalTs  TsampNgainVariant=Passthrough  TsampIntegralVariant=Disabled_SignalSpec  ExternalSaturationOutDataTypeStr=Inherit: Same as second input  DerivativeSourceVariant=ErrorSignal  PreIntVariant=InternalPreInt
      settings: LibrarySourceBlock=simulink/Discrete/Discrete PID Controller
  Gain{,1,4..5} (4 alike) : Gain
  Gain2 : Gain  Gain=-1
  Gain3 : Gain  Gain=-1
  Mux : Mux  Inputs=2
  Mux1 : Mux  Inputs=3
  Mux2 : Mux  Inputs=2
  Mux3 : Mux  Inputs=3
  Mux4 : Mux  Inputs=2
  Saturation : Saturate  UpperLimit=MaxAttitudeSetpoint  LowerLimit=-MaxAttitudeSetpoint
  Scope1 : Scope
      settings: ActiveDisplayYMinimum=-1.6411066157427356  ActiveDisplayYMaximum=2.7856703008085013  DataLoggingVariableName=ScopeData13
  Scope2 : Scope  NumInputPorts=2
      settings: ActiveDisplayYMinimum=-8.1662533850353878  ActiveDisplayYMaximum=1.0364100310625961  DataLoggingVariableName=ScopeData11
  Subtract : Sum  Inputs=+-
  Switch : Switch  Criteria=u2 > Threshold  Threshold=4  SaturateOnIntegerOverflow=off  InputSameDT=off
  Pitch Yaw Setpoint : Outport
  wires:
  Vel/1 -> Scope2/2
  Ascent Controller/1 -> Demux/1
  Pos/1 -> Subtract/1
  Setpoint Downrange CrossRange/1 -> Demux1/1
  Mux1/1 -> Subtract/2
  Gain/1 -> Mux/2
  Descent Controller/1 -> Demux2/1
  Mux2/1 -> Switch/1
  Mux/1 -> Switch/3
  Switch/1 -> Scope1/1, Saturation/1
  Clock/1 -> Switch/2
  Gain2/1 -> Mux/1
  Demux/2 -> Gain2/1
  Demux/3 -> Gain/1
  Demux2/2 -> Gain3/1
  Demux2/3 -> Gain1/1
  Subtract/1 -> Demux3/1
  Demux3/1 -> Mux3/1
  Mux3/1 -> Descent Controller/1, Ascent Controller/1
  Demux3/2 -> Gain4/1
  Gain4/1 -> Mux3/2
  Gain5/1 -> Mux3/3
  Demux3/3 -> Gain5/1
  Gain3/1 -> Mux2/1
  Gain1/1 -> Mux2/2
  Saturation/1 -> Demux4/1
  Demux4/1 -> Mux4/2
  Demux4/2 -> Mux4/1
  Mux4/1 -> Pitch Yaw Setpoint/1
  Demux1/1 -> Mux1/3
  Demux1/2 -> Mux1/2

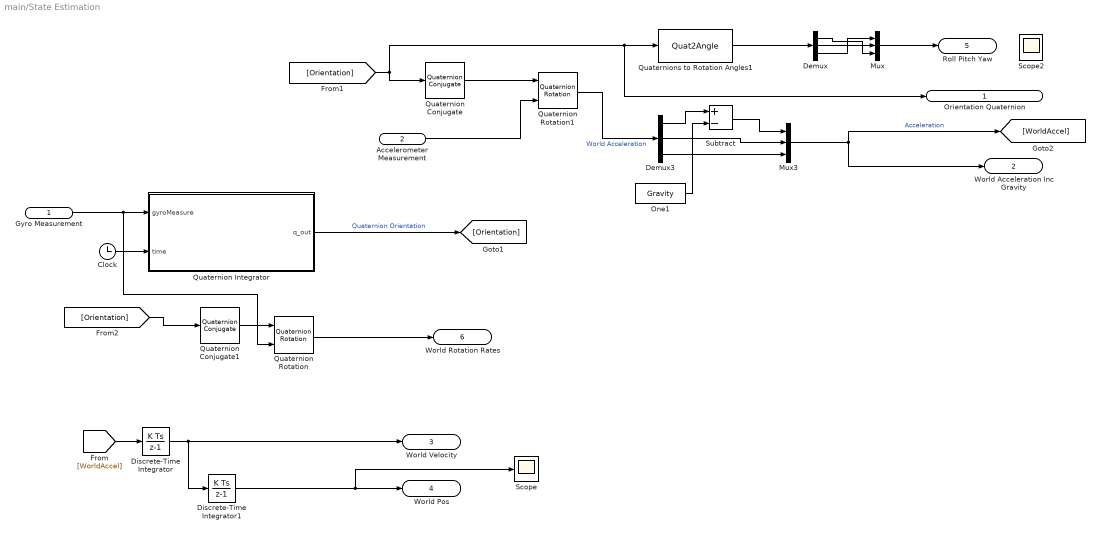
== system main/State Estimation ==
  Gyro Measurement : Inport
  Accelerometer Measurement : Inport  Port=2
  Clock : Clock
  Demux : Demux  Outputs=3
  Demux3 : Demux  Outputs=3
  Discrete-Time Integrator : DiscreteIntegrator  SampleTime=-1  ICPrevOutput=DiscIntNeverNeededParam  ICPrevScaledInput=DiscIntNeverNeededParam
  Discrete-Time Integrator1 : DiscreteIntegrator  SampleTime=-1  ICPrevOutput=DiscIntNeverNeededParam  ICPrevScaledInput=DiscIntNeverNeededParam
  Mux : Mux  Inputs=3
  Mux3 : Mux  Inputs=3
  One1 : Constant  Value=Gravity  OutDataTypeStr=Inherit: Inherit via back propagation
  Quaternion Conjugate : aerolibutil/Quaternion Conjugate
  Quaternion Conjugate1 : aerolibutil/Quaternion Conjugate
  Quaternion Rotation : aerolibutil/Quaternion Rotation
  Quaternion Rotation1 : aerolibutil/Quaternion Rotation
  Quaternion Integrator : MATLAB Function  TreatAsAtomicUnit=on
  Quaternions to Rotation Angles1 : Quat2Angle
      settings: AttributesFormatString=Rotation Order: %<rotationOrder>
  Scope : Scope
      settings: ActiveDisplayYMinimum=-210.62964690162914  ActiveDisplayYMaximum=885.29202465036917  DataLoggingVariableName=ScopeData20
  Scope2 : Scope  NumInputPorts=2
      settings: ActiveDisplayYMinimum=-0.186237948766744  ActiveDisplayYMaximum=-0.05303396772787948  DataLoggingVariableName=ScopeData22
  Subtract : Sum  Inputs=+-
  Orientation Quaternion : Outport  Unit=one
  World Acceleration Inc Gravity : Outport  Port=2  Unit=one
  World Velocity : Outport  Port=3  Unit=one
  World Pos : Outport  Port=4  Unit=one
  Roll Pitch Yaw : Outport  Port=5  Unit=rad
  World Rotation Rates : Outport  Port=6  Unit=rad
  wires:
  Clock/1 -> Quaternion Integrator/2(time)
  Gyro Measurement/1 -> Quaternion Rotation/2, Quaternion Integrator/1(gyroMeasure)
  Quaternion Integrator/1(q_out) -> [Orientation]  "Quaternion Orientation"
  [WorldAccel] -> Discrete-Time Integrator/1
  Discrete-Time Integrator/1 -> Discrete-Time Integrator1/1, World Velocity/1
  Discrete-Time Integrator1/1 -> Scope/1, World Pos/1
  [Orientation] -> Quaternion Conjugate/1, Orientation Quaternion/1, Quaternions to Rotation Angles1/1
  One1/1 -> Subtract/2
  Quaternion Rotation1/1 -> Demux3/1  "World Acceleration"
  Mux3/1 -> [WorldAccel], World Acceleration Inc Gravity/1  "Acceleration"
  Accelerometer Measurement/1 -> Quaternion Rotation1/2
  Demux3/1 -> Subtract/1
  Subtract/1 -> Mux3/1
  Mux/1 -> Roll Pitch Yaw/1
  Quaternions to Rotation Angles1/1 -> Demux/1
  Demux/3 -> Mux/1
  Demux/2 -> Mux/2
  Demux/1 -> Mux/3
  Demux3/2 -> Mux3/2
  Demux3/3 -> Mux3/3
  Quaternion Conjugate/1 -> Quaternion Rotation1/1
  [Orientation] -> Quaternion Conjugate1/1
  Quaternion Conjugate1/1 -> Quaternion Rotation/1
  Quaternion Rotation/1 -> World Rotation Rates/1

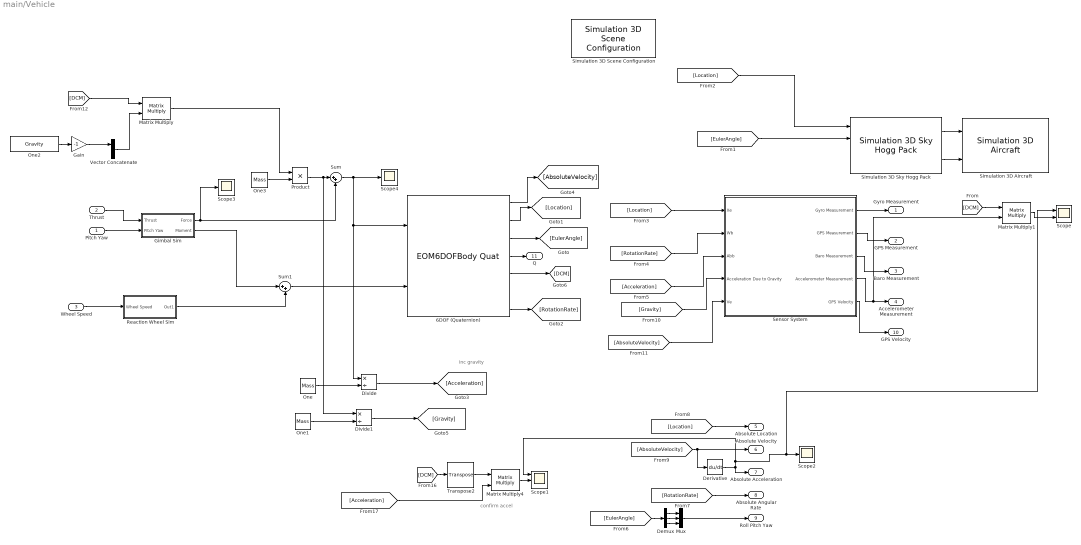
== system main/Vehicle ==
  note: confirm accel
  note: inc gravity
  Pitch Yaw : Inport
  Thrust : Inport  Port=2
  Wheel Speed : Inport  Port=3
  6DOF (Quaternion) : EOM6DOFBodyQuat  pm_0=[0.3 0.0 0.0]  mass_0=Mass  inertia=VehicleMOI
  Demux : Demux  Outputs=3
  Derivative : Derivative
  Divide : Product  Inputs=*/
  Divide1 : Product  Inputs=*/
  Gain : Gain  Gain=-1
  Gimbal Sim : Subsystem
  Matrix Multiply : Product  Multiplication=Matrix(*)
  Matrix Multiply1 : Product  Multiplication=Matrix(*)
  Matrix Multiply4 : Product  Multiplication=Matrix(*)
  Mux : Mux  Inputs=3
  One : Constant  Value=Mass  OutDataTypeStr=Inherit: Inherit via back propagation
  One1 : Constant  Value=Mass  OutDataTypeStr=Inherit: Inherit via back propagation
  One2 : Constant  Value=Gravity  OutDataTypeStr=Inherit: Inherit via back propagation
  One3 : Constant  Value=Mass  OutDataTypeStr=Inherit: Inherit via back propagation
  Product : Product
  Reaction Wheel Sim : Subsystem
  Scope : Scope  NumInputPorts=2
      settings: ActiveDisplayYMinimum=-2.1794175331295316  ActiveDisplayYMaximum=-1.4721698653540805  DataLoggingVariableName=ScopeData26
  Scope1 : Scope  NumInputPorts=3
      settings: TimeSpan=20  ActiveDisplayYMinimum=-13.628639838881007  ActiveDisplayYMaximum=17.495362789825904  DataLoggingVariableName=ScopeData18
  Scope2 : Scope
      settings: ActiveDisplayYMinimum=-0.23505611203130927  ActiveDisplayYMaximum=0.70157906130108261  DataLoggingVariableName=ScopeData19
  Scope3 : Scope
      settings: DataLoggingVariableName=ScopeData21
  Scope4 : Scope
      settings: ActiveDisplayYMinimum=-8.7926786300855966  ActiveDisplayYMaximum=9.3402291634712  DataLoggingVariableName=ScopeData25
  Sensor System : Subsystem
  Simulation 3D Aircraft : aerolibsim3d/Simulation 3D Aircraft  Priority=-1  Mesh=Sky Hogg  MeshPath=/MathWorksAerospaceContent/Vehicles/Aircraft/Custom/Mesh/SK_HL20.SK_HL20  MeshPathAT=/MathWorksAerospaceContent/Vehicles/Aircraft/AirTransport/Mesh/SK_AirTransport.SK_AirTransport  MeshPathGA=/MathWorksAerospaceContent/Vehicles/Aircraft/GeneralAviation/Mesh/SK_GeneralAviation.SK_GeneralAviation  AircraftColor=Red  ActorName=SimulinkVehicle3  Translation=zeros( 11, 3 )  Rotation=zeros( 11, 3 )  ScaleInputPort=Dialog  Scale=[1 1 1]  InitialScale=[1 1 1]  IsGHSensorEnabled=on  AreGHRaysVisible=off  IsOutputReshapeEnabled=off  GHRayLength=1524  GHBodyOffset=0.90  GHFrontTireRadius=0.21  GHLeftTireRadius=0.21  GHRightTireRadius=0.21  WoWSensorTolerance=0.05  LightsConfig=Automatic lights  LandingLightIntensity=300000  LandingLightConeAngle=15  CustomLeftLandingLightLocation=[0 0 0]  CustomLeftLandingLightOrientation=[0 0 0]  CustomRightLandingLightLocation=[0 0 0]  CustomRightLandingLightOrientation=[0 0 0]  TaxiLightIntensity=150000  TaxiLightConeAngle=36  CustomTaxiLightLocation=[0 0 0]  CustomTaxiLightOrientation=[0 0 0]  NavLightIntensity=500  PositionLightIntensity=500  StrobeLightIntensity=5000  WingtipStrobePeriod=1.5  WingtipStrobePulseWidth=6  TailStrobePeriod=1.5  TailStrobePulseWidth=6  BeaconLightIntensity=4000  BeaconPeriod=1.5  BeaconPulseWidth=10  SampleTime=-1  ActorType=SimulinkVehicle  ID=3  aMode=0  ActorTag=SimulinkVehicle3
  Simulation 3D Scene Configuration : sim3dlib/Simulation 3D Scene Configuration  Priority=0  ProjectFormat=Default Scenes  SceneDesc=Airport  ProjectName=C:\Program Files\MATLAB\R2025a\toolbox\shared\sim3d_projects\automotive_project_windows\UE\WindowsNoEditor\VehicleSimulation.exe  ScenePath=/Game/Maps/HwStrght  EnableOpenDRIVE=off  vehTagList={'Custom';'Scene Origin';'SimulinkVehicle3'}  vehTag=Custom  AttachedCameraRelativeTranslation=[0 0 0]  FreeCameraDefaultInitialTranslation=[-6, 0, 2]  AttachedCameraRelativeRotation=[0 0 0]  FreeCameraDefaultInitialRotation=[0, -15, 0]  ViewpointName=Custom  FreeCameraInitialTranslation=[-6 0 2]  ViewpointTranslation=[0 0 0]  FreeCameraInitialRotation=[0 0 0]  ViewpointRotation=[0 0 0]  OpVisEn=off  Ts=.02  EnableWindow=on  EnableRemoteAccess=off  EnableWeather=off  SunAzimuth=90  SunAltitude=40.0  EnableGeospatialSun=off  Latitude=0  Longitude=0  Date=2023-01-01  Time=10:30:00  GeoTimeZone=-5.0  SunDaylightSaving=off  wind=1  clouds=10  EnableVolumetricClouds=off  CloudCoverage=0  CloudAltitude=6  fog=0  rain=0  RaindropsEffect=off  SnowDensity=0  EnableGeospatial=off  TilesetSource=Earth terrain  UseTrueOrigin=off  OriginHeight=200  OriginLatitude=40.744652  OriginLongitude=-73.988864  MapStyle=Aerial  AdditionalAssetIDs=[]  UseAdvancedSunSky=off  SolarTime=11  TimeZone=-5  Day=21  Month=9  Year=2022  UseDaylightSavingTime=on  DSTStartDay=10  DSTStartMonth=3  DSTEndDay=3  DSTEndMonth=11  DSTSwitchHour=2  sensorTag=MainCamera2  sensorId=2  sensorName=MainCamera2  mountLoc=Origin  offsetFlag=off  tmountOffset=[0, 0, 0]  rmountOffset=[0, 0, 0]  HorizontalResolution=1280  VerticalResolution=720  HorizontalFOV=60  mountPoint=[0 0 0]  mountOrientation=[0 0 0]  aMode=0  ID=2  GeoTrigger=Inactive  ViewNameList={'Custom'}  ViewTranslationList={'[-6 0 2]'}  ViewRotationList={'[0 0 0]'}
      settings: AttributesFormatString=NED  LibrarySourceBlock=aerolibsim3d/Simulation 3D Scene Configuration
  Simulation 3D Sky Hogg Pack : aerolibsim3d/Simulation 3D Sky Hogg Pack  Propeller_R=off  Rudder_R=on  Elevator_R=on  Left_Aileron_R=off  Right_Aileron_R=off  Flaps_R=off  Nose_Wheel_Strut_R=off  Nose_Wheel_R=off  Left_Wheel_R=off  Right_Wheel_R=off  GeoRadioButton=NED
      settings: AttributesFormatString=NED
  Sum : Sum  Inputs=|++
  Sum1 : Sum  Inputs=|++
  Transpose2 : matrix_library/Transpose
  Vector Concatenate : Concatenate  NumInputs=3
  Gyro Measurement : Outport  Unit=rad/s  PortDimensions=3
  GPS Measurement : Outport  Port=2  Unit=m  PortDimensions=3
  Baro Measurement : Outport  Port=3  Unit=m  PortDimensions=1
  Accelerometer Measurement : Outport  Port=4  Unit=m/s^2  PortDimensions=3
  Absolute Location : Outport  Port=5  Unit=m  PortDimensions=3
  Absolute Velocity : Outport  Port=6  Unit=m/s  PortDimensions=3
  Absolute Acceleration : Outport  Port=7  Unit=m/s^2  PortDimensions=3
  Absolute Angular Rate : Outport  Port=8  Unit=rad/s  PortDimensions=3
  Roll Pitch Yaw : Outport  Port=9  Unit=rad  PortDimensions=3
  GPS Velocity : Outport  Port=10  Unit=m/s^2  PortDimensions=3
  Q : Outport  Port=11  Unit=rad/s
  wires:
  6DOF (Quaternion)/3 -> [EulerAngle]
  Gimbal Sim/1(Force) -> Scope3/1, Sum/2
  Sum/1 -> 6DOF (Quaternion)/1, Divide/1, Scope4/1
  Pitch Yaw/1 -> Gimbal Sim/2(Pitch Yaw)
  Thrust/1 -> Gimbal Sim/1(Thrust)
  6DOF (Quaternion)/2 -> [Location]
  [Location] -> Sensor System/1(Xe)
  6DOF (Quaternion)/7 -> [RotationRate]
  [RotationRate] -> Sensor System/2(Wb)
  [Acceleration] -> Sensor System/3(Abb)
  One/1 -> Divide/2
  Divide/1 -> [Acceleration]
  Sensor System/1(Gyro Measurement) -> Gyro Measurement/1
  Sensor System/2(GPS Measurement) -> GPS Measurement/1
  Sensor System/3(Baro Measurement) -> Baro Measurement/1
  Sensor System/4(Accelerometer Measurement) -> Matrix Multiply1/2, Accelerometer Measurement/1
  [RotationRate] -> Absolute Angular Rate/1
  [Location] -> Absolute Location/1
  6DOF (Quaternion)/1 -> [AbsoluteVelocity]
  [AbsoluteVelocity] -> Absolute Velocity/1, Derivative/1
  One1/1 -> Divide1/2
  Divide1/1 -> [Gravity]
  [Gravity] -> Sensor System/4(Acceleration Due to Gravity)
  [AbsoluteVelocity] -> Sensor System/5(Ve)
  Sensor System/5(GPS Velocity) -> GPS Velocity/1
  Wheel Speed/1 -> Reaction Wheel Sim/1(Wheel Speed)
  Reaction Wheel Sim/1(Out1) -> Sum1/2
  6DOF (Quaternion)/5 -> [DCM]
  Vector Concatenate/1 -> Matrix Multiply/2
  Product/1 -> Sum/1, Divide1/1
  One3/1 -> Product/2
  Demux/3 -> Mux/3
  [EulerAngle] -> Demux/1
  Mux/1 -> Roll Pitch Yaw/1
  Simulation 3D Sky Hogg Pack/1 -> Simulation 3D Aircraft/1
  Simulation 3D Sky Hogg Pack/2 -> Simulation 3D Aircraft/2
  [Location] -> Simulation 3D Sky Hogg Pack/1
  Sum1/1 -> 6DOF (Quaternion)/2
  [DCM] -> Matrix Multiply/1
  Matrix Multiply/1 -> Product/1
  [EulerAngle] -> Simulation 3D Sky Hogg Pack/2
  One2/1 -> Gain/1
  Gain/1 -> Vector Concatenate/1
  Demux/1 -> Mux/1
  Demux/2 -> Mux/2
  6DOF (Quaternion)/4 -> Q/1
  [DCM] -> Matrix Multiply1/1
  Matrix Multiply1/1 -> Scope/2
  Derivative/1 -> Scope1/1, Scope/1, Scope2/1, Absolute Acceleration/1
  [DCM] -> Transpose2/1
  Transpose2/1 -> Matrix Multiply4/1
  [Acceleration] -> Matrix Multiply4/2
  Matrix Multiply4/1 -> Scope1/2
  Gimbal Sim/2(Moment) -> Sum1/1

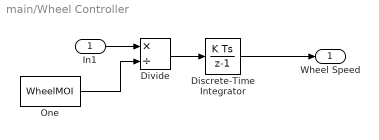
== system main/Wheel Controller ==
  In1 : Inport
  Discrete-Time Integrator : DiscreteIntegrator  SampleTime=-1  ICPrevOutput=DiscIntNeverNeededParam  ICPrevScaledInput=DiscIntNeverNeededParam
  Divide : Product  Inputs=*/
  One : Constant  Value=WheelMOI  OutDataTypeStr=Inherit: Inherit via back propagation
  Wheel Speed : Outport
  wires:
  In1/1 -> Divide/1
  One/1 -> Divide/2
  Divide/1 -> Discrete-Time Integrator/1
  Discrete-Time Integrator/1 -> Wheel Speed/1

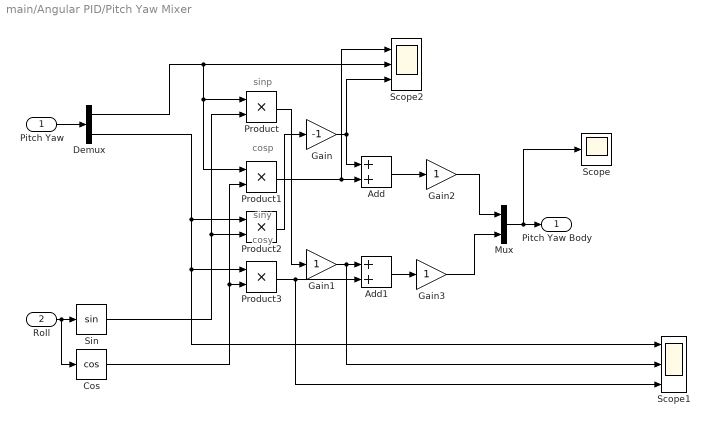
== system main/Angular PID/Pitch Yaw Mixer ==
  note: siny
  note: cosp
  note: cosy
  note: sinp
  Pitch Yaw : Inport
  Roll : Inport  Port=2
  Add : Sum
  Add1 : Sum
  Cos : Trigonometry  Operator=cos
  Demux : Demux  Outputs=2
  Gain : Gain  Gain=-1
  Gain1 : Gain
  Gain2 : Gain
  Gain3 : Gain
  Mux : Mux  Inputs=2
  Product{,1..3} (4 alike) : Product
  Scope : Scope
      settings: ActiveDisplayYMinimum=-4.9736350552420738  ActiveDisplayYMaximum=6.7199507264866654  DataLoggingVariableName=ScopeData10
  Scope1 : Scope  NumInputPorts=3
      settings: ActiveDisplayYMinimum=-0.19881934513771  ActiveDisplayYMaximum=0.18743086156856115  DataLoggingVariableName=ScopeData23
  Scope2 : Scope  NumInputPorts=3
      settings: ActiveDisplayYMinimum=-0.19881934513771  ActiveDisplayYMaximum=0.18743086156856115  DataLoggingVariableName=ScopeData24
  Sin : Trigonometry
  Pitch Yaw Body : Outport
  wires:
  Roll/1 -> Cos/1, Sin/1
  Mux/1 -> Scope/1, Pitch Yaw Body/1
  Sin/1 -> Product2/2, Product/2
  Cos/1 -> Product3/2, Product1/2
  Demux/2 -> Scope1/1, Product3/1, Product2/1
  Product1/1 -> Scope2/1, Add/2
  Product2/1 -> Gain/1
  Product3/1 -> Scope1/3, Add1/2
  Product/1 -> Gain1/1
  Gain1/1 -> Scope1/2, Add1/1
  Add/1 -> Gain2/1
  Add1/1 -> Gain3/1
  Gain3/1 -> Mux/2
  Gain2/1 -> Mux/1
  Gain/1 -> Scope2/3, Add/1
  Pitch Yaw/1 -> Demux/1
  Demux/1 -> Product1/1, Product/1, Scope2/2

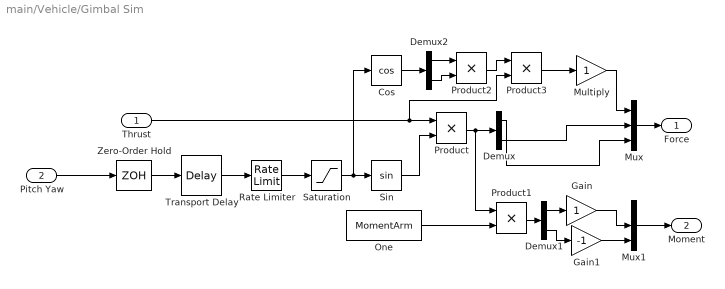
== system main/Vehicle/Gimbal Sim ==
  Thrust : Inport  PortDimensions=1
  Pitch Yaw : Inport  Port=2  PortDimensions=2
  Cos : Trigonometry  Operator=cos
  Demux : Demux  Outputs=2
  Demux1 : Demux  Outputs=2
  Demux2 : Demux  Outputs=2
  Gain : Gain
  Gain1 : Gain  Gain=-1
  Multiply : Gain
  Mux : Mux  Inputs=3
  Mux1 : Mux  Inputs=3
  One : Constant  Value=MomentArm  OutDataTypeStr=Inherit: Inherit via back propagation
  Product{,1..3} (4 alike) : Product
  Rate Limiter : RateLimiter  RisingSlewLimit=GimbalMaxRate  FallingSlewLimit=-GimbalMaxRate  SampleTimeMode=inherited
  Saturation : Saturate  UpperLimit=GimbalMaxSkew  LowerLimit=-GimbalMaxSkew
  Sin : Trigonometry
  Transport Delay : TransportDelay  DelayTime=GimbalDelay
  Zero-Order Hold : ZeroOrderHold  SampleTime=ServoSampleTime
  Force : Outport
  Moment : Outport  Port=2
  wires:
  Pitch Yaw/1 -> Zero-Order Hold/1
  Transport Delay/1 -> Rate Limiter/1
  Rate Limiter/1 -> Saturation/1
  Saturation/1 -> Cos/1, Sin/1
  Sin/1 -> Product/2
  Mux/1 -> Force/1
  Thrust/1 -> Product3/2, Product/1
  Product/1 -> Product1/1, Demux/1
  Product1/1 -> Demux1/1
  One/1 -> Product1/2
  Mux1/1 -> Moment/1
  Cos/1 -> Demux2/1
  Demux2/1 -> Product2/1
  Demux2/2 -> Product2/2
  Product2/1 -> Product3/1
  Product3/1 -> Multiply/1
  Zero-Order Hold/1 -> Transport Delay/1
  Demux1/1 -> Gain/1
  Gain/1 -> Mux1/2
  Demux1/2 -> Gain1/1
  Gain1/1 -> Mux1/3
  Multiply/1 -> Mux/1
  Demux/2 -> Mux/2
  Demux/1 -> Mux/3

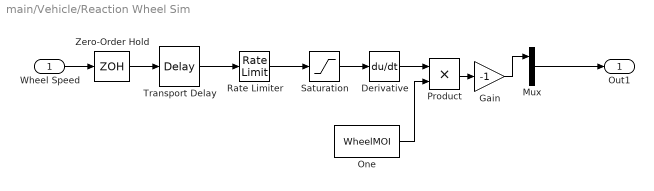
== system main/Vehicle/Reaction Wheel Sim ==
  Wheel Speed : Inport
  Derivative : Derivative
  Gain : Gain  Gain=-1
  Mux : Mux  Inputs=3
  One : Constant  Value=WheelMOI  OutDataTypeStr=Inherit: Inherit via back propagation
  Product : Product
  Rate Limiter : RateLimiter  RisingSlewLimit=WheelMaxAcceleration  FallingSlewLimit=-WheelMaxAcceleration  SampleTimeMode=inherited
  Saturation : Saturate  UpperLimit=WheelMaxRate  LowerLimit=-WheelMaxRate
  Transport Delay : TransportDelay  DelayTime=WheelDelay
  Zero-Order Hold : ZeroOrderHold  SampleTime=WheelSampleTime
  Out1 : Outport
  wires:
  Wheel Speed/1 -> Zero-Order Hold/1
  Transport Delay/1 -> Rate Limiter/1
  Zero-Order Hold/1 -> Transport Delay/1
  Rate Limiter/1 -> Saturation/1
  Saturation/1 -> Derivative/1
  Derivative/1 -> Product/1
  One/1 -> Product/2
  Product/1 -> Gain/1
  Mux/1 -> Out1/1
  Gain/1 -> Mux/1

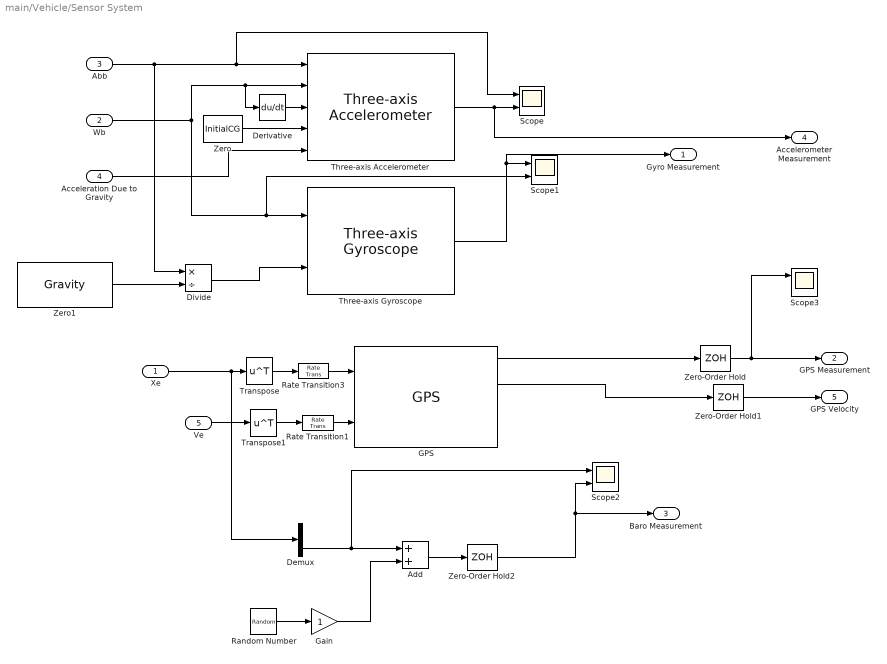
== system main/Vehicle/Sensor System ==
  Xe : Inport  Unit=m
  Wb : Inport  Port=2  Unit=rad/s  PortDimensions=3
  Abb : Inport  Port=3  Unit=m/s^2  PortDimensions=3
  Acceleration Due to Gravity : Inport  Port=4  Unit=m/s^2  PortDimensions=3
  Ve : Inport  Port=5  Unit=m/s
  Add : Sum
  Demux : Demux  Outputs=3
  Derivative : Derivative
  Divide : Product  Inputs=*/
  GPS : sensorgpslib/GPS  DispRefFrame=NED  PositionInputFormat=Local  ReferenceLocation=[ 0, 0, 0 ]  HorizontalPositionAccuracy=0.01  VerticalPositionAccuracy=0.01  VelocityAccuracy=0.05  DecayFactor=0.999  SeedDouble=67  SimulateUsing=Interpreted execution
      settings: LibrarySourceBlock=mspsensorlib/GPS
  Gain : Gain
  Random Number : RandomNumber  Variance=0.1  SampleTime=BaroSampleTime
  Rate Transition1 : RateTransition  OutPortSampleTime=.01
  Rate Transition3 : RateTransition  OutPortSampleTime=.01
  Scope{,1..3} (4 alike) : Scope  NumInputPorts=2
      Scope settings: ActiveDisplayYMinimum=-2.7229097693980622  ActiveDisplayYMaximum=2.0923322147247863
      Scope1 settings: ActiveDisplayYMinimum=-0.022041845758303483  ActiveDisplayYMaximum=0.045884895263552071
      Scope2 settings: ActiveDisplayYMinimum=-2.4626226622119756  ActiveDisplayYMaximum=1.2147011299910595
      Scope3 settings: ActiveDisplayYMinimum=-3.8365102675467204  ActiveDisplayYMaximum=33.227966829817731  DataLoggingVariableName=ScopeData2
  Three-axis Accelerometer : aerolibnav/Three-axis Accelerometer  units=Metric (MKS)  acc=IMULocation  gtype=on  dtype_a=on  w_a=190  z_a=0.707  a_sf_cc=[1 0 0; 0 1 0; 0 0 1]  a_bias=[0 0 0]  a_Ts=AccelSampleTime  a_rand=off  a_seeds=[23093 23094 23095]  a_pow=AccelNoise  a_sat="[-inf  -inf  -inf  inf inf inf]"
  Three-axis Gyroscope : aerolibnav/Three-axis Gyroscope  dtype_g=on  w_g=190  z_g=0.707  g_sf_cc=[1 0 0; 0 1 0; 0 0 1]  g_bias=[0 0 0]  g_sen=[0 0 0]  g_Ts=GyroSampleTime  g_rand=off  g_seeds=[23093 23094 23095]  g_pow=GyroNoise  g_sat="[-inf  -inf  -inf  inf inf inf]"
  Transpose : Math  Operator=transpose
  Transpose1 : Math  Operator=transpose
  Zero : Constant  Value=InitialCG  OutDataTypeStr=Inherit: Inherit via back propagation
  Zero-Order Hold : ZeroOrderHold  SampleTime=GPSSampleTime
  Zero-Order Hold1 : ZeroOrderHold  SampleTime=GPSSampleTime
  Zero-Order Hold2 : ZeroOrderHold  SampleTime=BaroSampleTime
  Zero1 : Constant  Value=Gravity  OutDataTypeStr=Inherit: Inherit via back propagation
  Gyro Measurement : Outport
  GPS Measurement : Outport  Port=2
  Baro Measurement : Outport  Port=3
  Accelerometer Measurement : Outport  Port=4
  GPS Velocity : Outport  Port=5
  wires:
  Wb/1 -> Derivative/1, Three-axis Accelerometer/2, Scope1/2, Three-axis Gyroscope/1
  Zero/1 -> Three-axis Accelerometer/4
  Abb/1 -> Divide/1, Scope/1, Three-axis Accelerometer/1
  Derivative/1 -> Three-axis Accelerometer/3
  Three-axis Accelerometer/1 -> Accelerometer Measurement/1, Scope/2
  Zero1/1 -> Divide/2
  Three-axis Gyroscope/1 -> Gyro Measurement/1, Scope1/1
  Divide/1 -> Three-axis Gyroscope/2
  Xe/1 -> Transpose/1, Demux/1
  Zero-Order Hold/1 -> Scope3/1, GPS Measurement/1
  Zero-Order Hold1/1 -> GPS Velocity/1
  Add/1 -> Zero-Order Hold2/1
  Random Number/1 -> Gain/1
  Gain/1 -> Add/2
  Demux/3 -> Scope2/1, Add/1
  Zero-Order Hold2/1 -> Scope2/2, Baro Measurement/1
  Transpose/1 -> Rate Transition3/1
  Transpose1/1 -> Rate Transition1/1
  Ve/1 -> Transpose1/1
  Rate Transition3/1 -> GPS/1
  Rate Transition1/1 -> GPS/2
  GPS/1 -> Zero-Order Hold/1
  GPS/2 -> Zero-Order Hold1/1
  Acceleration Due to Gravity/1 -> Three-axis Accelerometer/5
